simulink subsystem "RoboRio_Controls_sub"  (R2023b)
settings: Solver=VariableStepAuto  StartTime=0.0  StopTime=10.0  RelTol=1e-3
libraries: Autonomous_lib x1, Disabled_lib x1, Teleop_lib x1, Test_lib x1
settings Model: Creator=USER  LastModifiedBy=ander

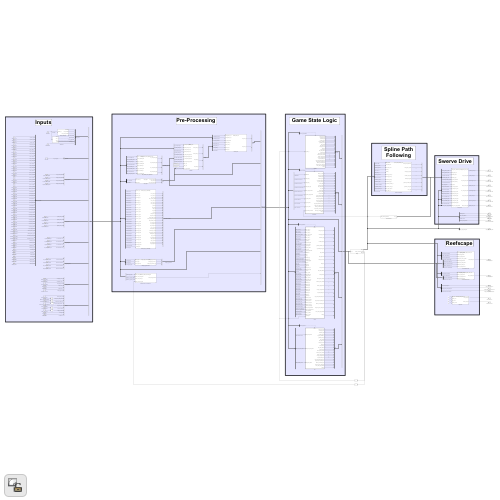
[thumbnail: Simulink's stored preview of the top-level diagram]
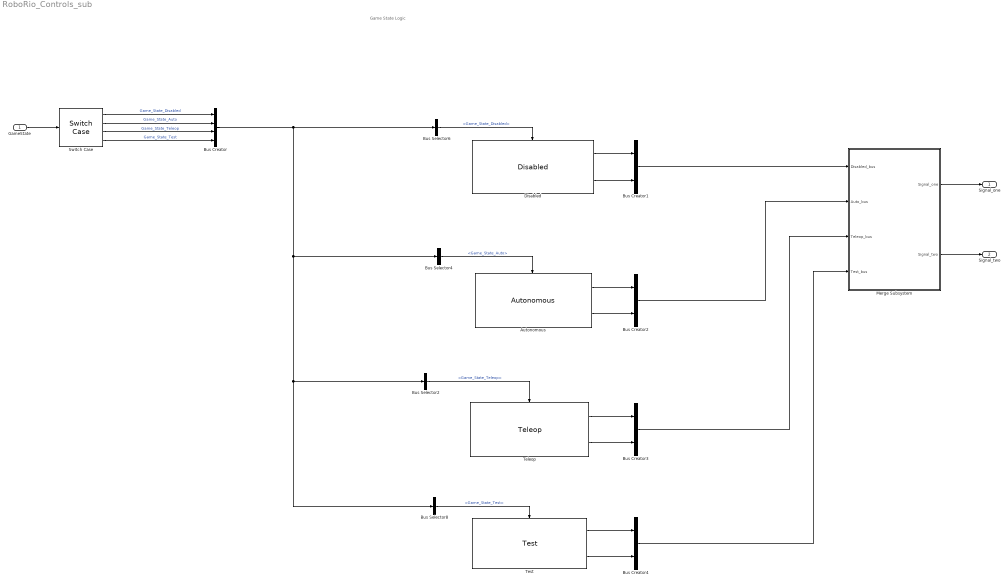
== system RoboRio_Controls_sub ==
  note: Game State Logic
  GameState : Inport
  Autonomous : Autonomous_lib/Autonomous  SystemSampleTime=-1  VariantActivationTime=update diagram  AllowFlexibleInterface=on  Latency=0  AutoFrameSizeCalculation=off
  Bus Creator : BusCreator  Inputs=4
  Bus Creator{1..4} (4 alike) : BusCreator  Inputs=2
  Bus Selector2 : BusSelector  OutputSignals=Game_State_Teleop
  Bus Selector4 : BusSelector  OutputSignals=Game_State_Auto
  Bus Selector6 : BusSelector  OutputSignals=Game_State_Disabled
  Bus Selector8 : BusSelector  OutputSignals=Game_State_Test
  Disabled : Disabled_lib/Disabled  SystemSampleTime=-1  VariantActivationTime=update diagram  AllowFlexibleInterface=on  Latency=0  AutoFrameSizeCalculation=off
  Merge Subsystem : Subsystem
  Switch Case : SwitchCase  CaseConditions={0,1,2}
  Teleop : Teleop_lib/Teleop  SystemSampleTime=-1  VariantActivationTime=update diagram  AllowFlexibleInterface=on  Latency=0  AutoFrameSizeCalculation=off
  Test : Test_lib/Test  SystemSampleTime=-1  VariantActivationTime=update diagram  AllowFlexibleInterface=on  Latency=0  AutoFrameSizeCalculation=off
  Signal_one : Outport
  Signal_two : Outport  Port=2
  wires:
  Bus Selector2/1 -> Teleop/Action  "<Game_State_Teleop>"
  Bus Selector4/1 -> Autonomous/Action  "<Game_State_Auto>"
  Bus Selector6/1 -> Disabled/Action  "<Game_State_Disabled>"
  Bus Selector8/1 -> Test/Action  "<Game_State_Test>"
  GameState/1 -> Switch Case/1
  Switch Case/1 -> Bus Creator/1  "Game_State_Disabled"
  Switch Case/2 -> Bus Creator/2  "Game_State_Auto"
  Switch Case/3 -> Bus Creator/3  "Game_State_Teleop"
  Switch Case/4 -> Bus Creator/4  "Game_State_Test"
  Bus Creator/1 -> Bus Selector6/1, Bus Selector4/1, Bus Selector2/1, Bus Selector8/1
  Disabled/1 -> Bus Creator1/1
  Disabled/2 -> Bus Creator1/2
  Autonomous/1 -> Bus Creator2/1
  Autonomous/2 -> Bus Creator2/2
  Teleop/1 -> Bus Creator3/1
  Teleop/2 -> Bus Creator3/2
  Test/1 -> Bus Creator4/1
  Test/2 -> Bus Creator4/2
  Bus Creator1/1 -> Merge Subsystem/1(Disabled_bus)
  Bus Creator2/1 -> Merge Subsystem/2(Auto_bus)
  Bus Creator3/1 -> Merge Subsystem/3(Teleop_bus)
  Bus Creator4/1 -> Merge Subsystem/4(Test_bus)
  Merge Subsystem/1(Signal_one) -> Signal_one/1
  Merge Subsystem/2(Signal_two) -> Signal_two/1

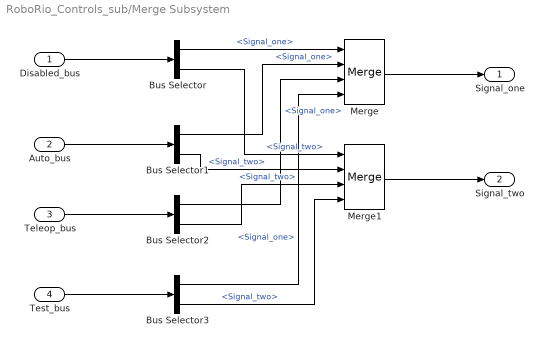
== system RoboRio_Controls_sub/Merge Subsystem ==
  Disabled_bus : Inport
  Auto_bus : Inport  Port=2
  Teleop_bus : Inport  Port=3
  Test_bus : Inport  Port=4
  Bus Selector{,1..3} (4 alike) : BusSelector  OutputSignals=Signal_one,Signal_two
  Merge : Merge  Inputs=4
  Merge1 : Merge  Inputs=4
  Signal_one : Outport
  Signal_two : Outport  Port=2
  wires:
  Bus Selector3/2 -> Merge1/4  "<Signal_two>"
  Bus Selector2/2 -> Merge1/3  "<Signal_two>"
  Bus Selector1/2 -> Merge1/2  "<Signal_two>"
  Bus Selector/2 -> Merge1/1  "<Signal_two>"
  Merge1/1 -> Signal_two/1
  Merge/1 -> Signal_one/1
  Bus Selector3/1 -> Merge/4  "<Signal_one>"
  Bus Selector2/1 -> Merge/3  "<Signal_one>"
  Bus Selector1/1 -> Merge/2  "<Signal_one>"
  Bus Selector/1 -> Merge/1  "<Signal_one>"
  Test_bus/1 -> Bus Selector3/1
  Teleop_bus/1 -> Bus Selector2/1
  Auto_bus/1 -> Bus Selector1/1
  Disabled_bus/1 -> Bus Selector/1
